simulink model "SDEC_Motor_Model"  (R2024b)
settings: Solver=VariableStepAuto  StartTime=0.0  StopTime=10.0  RelTol=1e-3
values from neighbouring files (symbols this model uses):
  Kphi = 1.6    [SEDC_motor.m]
  TL = 20    [SEDC_motor.m]
  Va = 160    [SEDC_motor.m]
settings Model: Creator=Ahmad  LastModifiedBy=Ahmad

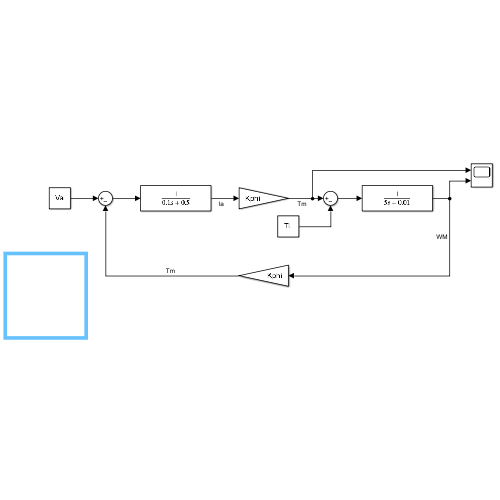
[thumbnail: Simulink's stored preview of the top-level diagram]
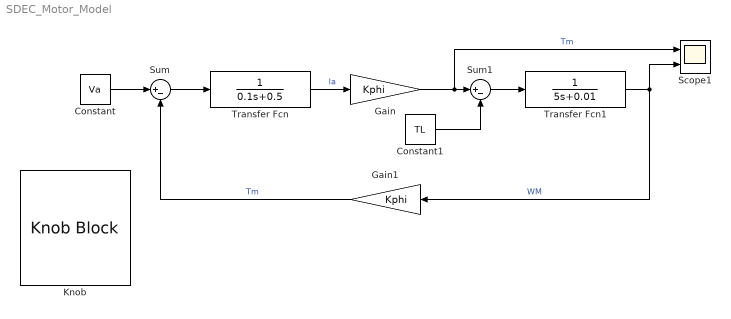
== system SDEC_Motor_Model ==
  Constant : Constant  Value=Va
  Constant1 : Constant  Value=TL
  Gain : Gain  Gain=Kphi
  Gain1 : Gain  Gain=Kphi
  Knob : KnobBlock
  Scope1 : Scope  NumInputPorts=2
  Sum : Sum  Inputs=|+-
  Sum1 : Sum  Inputs=|+-
  Transfer Fcn : TransferFcn  Denominator=[0.1, 0.5]
  Transfer Fcn1 : TransferFcn  Denominator=[5, 0.01]
  wires:
  Constant/1 -> Sum/1
  Sum/1 -> Transfer Fcn/1
  Transfer Fcn/1 -> Gain/1  "la"
  Gain/1 -> Scope1/1, Sum1/1  "Tm"
  Constant1/1 -> Sum1/2
  Sum1/1 -> Transfer Fcn1/1
  Gain1/1 -> Sum/2  "Tm"
  Transfer Fcn1/1 -> Scope1/2, Gain1/1  "WM"
